simulink model "dyn_model"  (R2016b)
settings: Solver=VariableStepAuto  StartTime=0.0  StopTime=20  RelTol=1e-3
undefined symbols (not defined in the file or in its folder): D1, Delta
libraries: powerlib x29
settings Model: SimulationMode=accelerator  Creator=tinrabuzin  LastModifiedBy=tinrabuzin
settings SolverCC: ZeroCrossAlgorithm=Adaptive
settings DebuggingCC: UnconnectedInputMsg=none  UnconnectedOutputMsg=none  UnconnectedLineMsg=none

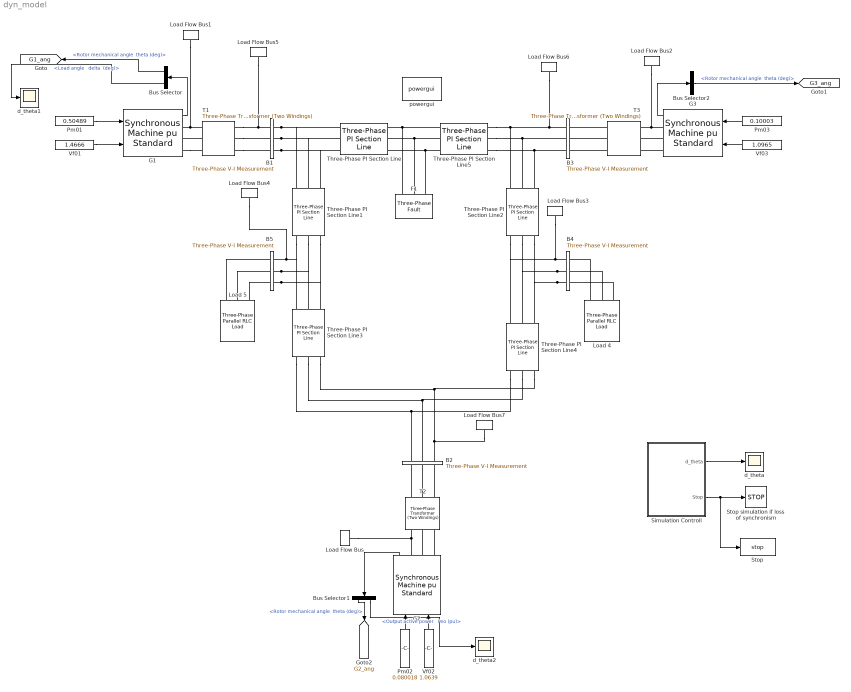
== system dyn_model ==
  B1 : powerlib/Measurements/Three-Phase V-I Measurement  VoltageMeasurement=phase-to-ground  SetLabelV=on  LabelV=Vabc_B1  Vpu=off  VpuLL=off  CurrentMeasurement=yes  SetLabelI=on  LabelI=Iabc_B1  Ipu=off  Pbase=100e6  Vbase=500e3  OutputType=Complex  PhasorSimulation=on  PSBequivalent=0
  B2 : powerlib/Measurements/Three-Phase V-I Measurement  VoltageMeasurement=phase-to-ground  SetLabelV=on  LabelV=Vabc_B2  Vpu=off  VpuLL=off  CurrentMeasurement=yes  SetLabelI=on  LabelI=Iabc_B2  Ipu=off  Pbase=100e6  Vbase=500e3  OutputType=Complex  PhasorSimulation=on  PSBequivalent=0
  B3 : powerlib/Measurements/Three-Phase V-I Measurement  VoltageMeasurement=phase-to-ground  SetLabelV=on  LabelV=Vabc_B3  Vpu=off  VpuLL=off  CurrentMeasurement=yes  SetLabelI=on  LabelI=Iabc_B3  Ipu=off  Pbase=100e6  Vbase=500e3  OutputType=Complex  PhasorSimulation=on  PSBequivalent=0
  B4 : powerlib/Measurements/Three-Phase V-I Measurement  VoltageMeasurement=phase-to-ground  SetLabelV=on  LabelV=Vabc_B4  Vpu=off  VpuLL=off  CurrentMeasurement=yes  SetLabelI=on  LabelI=Iabc_B4  Ipu=off  Pbase=100e6  Vbase=500e3  OutputType=Complex  PhasorSimulation=on  PSBequivalent=0
  B5 : powerlib/Measurements/Three-Phase V-I Measurement  VoltageMeasurement=phase-to-ground  SetLabelV=on  LabelV=Vabc_B5  Vpu=off  VpuLL=off  CurrentMeasurement=yes  SetLabelI=on  LabelI=Iabc_B5  Ipu=off  Pbase=100e6  Vbase=500e3  OutputType=Complex  PhasorSimulation=on  PSBequivalent=0
  Bus Selector : BusSelector  OutputSignals="Mechanical.Rotor mechanical angle  theta (deg),Load angle   delta  (deg)"
  Bus Selector1 : BusSelector  OutputSignals="Mechanical.Rotor mechanical angle  theta (deg),Output active power   Peo (pu)"
  Bus Selector2 : BusSelector  OutputSignals="Mechanical.Rotor mechanical angle  theta (deg)"
  F1 : powerlib/Elements/Three-Phase Fault  InitialStates=0  FaultA=on  FaultB=on  FaultC=on  GroundFault=on  SwitchTimes=[1 4.5005]  External=off  SwitchStatus=NaN  FaultResistance=0.0001  GroundResistance=0.0001  SnubberResistance=1e6  SnubberCapacitance=inf  Measurements=None
  G1 : powerlib/Machines/Synchronous Machine pu Standard  PresetModel=No  MechanicalLoad=Mechanical power Pm  ShowDetailedParameters=on  RotorType=Round  Units=per unit standard parameters  MeasurementBus=off  NominalParameters="[200E6  24000   50 ]"  Reactances1=[1.8 .3 .25 1.7 .55 .25 .2]  Reactances2=[ 1.305, 0.296, 0.252, 0.474, 0.243, 0.18 ]  dAxisTimeConstants=Open-circuit  qAxisTimeConstants=Open-circuit  TimeConstants1=[]  TimeConstants2=[8 .03 .4 .05]  TimeConstants3=[]  TimeConstants4=[]  TimeConstants5=[ 1.01, 0.053, 0.1 ]  TimeConstants6=[]  TimeConstants7=[]  TimeConstants8=[]  StatorResistance=0.0025  Mechanical=[ 6.5 0 2]  PolePairs=4  InitialConditions=[0 -53.1702 0.511213 0.511213 0.511213 -9.47522 -129.475 110.525 1.46662]  SetSaturation=off  Saturation=[0.6404,0.7127,0.8441,0.9214,0.9956,1.082,1.19,1.316,1.457;0.7,0.7698,0.8872,0.9466,0.9969,1.046,1.1,1.151,1.201]  LoadFlowParameters=[2 700000000 0 0 0]  TsPowergui=0  TsBlock=-1  IterativeModel=Trapezoidal non iterative  IterativeDiscreteModel=Trapezoidal non iterative  BusType=swing  Pref=700000000  Qref=0  Qmin=-Inf  Qmax=Inf  PLF=0  QLF=0
      settings: AttributesFormatString=\n\n
  G2 : powerlib/Machines/Synchronous Machine pu Standard  PresetModel=No  MechanicalLoad=Mechanical power Pm  ShowDetailedParameters=on  RotorType=Round  Units=per unit standard parameters  MeasurementBus=off  NominalParameters="[200E6  24000   50 ]"  Reactances1=[1.8 .3 .25 1.7 .55 .25 .2]  Reactances2=[ 1.305, 0.296, 0.252, 0.474, 0.243, 0.18 ]  dAxisTimeConstants=Open-circuit  qAxisTimeConstants=Open-circuit  TimeConstants1=[]  TimeConstants2=[8 .03 .4 .05]  TimeConstants3=[]  TimeConstants4=[]  TimeConstants5=[ 1.01, 0.053, 0.1 ]  TimeConstants6=[]  TimeConstants7=[]  TimeConstants8=[]  StatorResistance=0.0025  Mechanical=[ 6.5 0 2]  PolePairs=4  InitialConditions=[0 -91.9476 0.0854428 0.0854428 0.0854428 -29.8718 -149.872 90.1282 1.06392]  SetSaturation=off  Saturation=[0.6404,0.7127,0.8441,0.9214,0.9956,1.082,1.19,1.316,1.457;0.7,0.7698,0.8872,0.9466,0.9969,1.046,1.1,1.151,1.201]  LoadFlowParameters=[1 700000000 0 0 0]  TsPowergui=0  TsBlock=-1  IterativeModel=Trapezoidal non iterative  IterativeDiscreteModel=Trapezoidal non iterative  BusType=PQ  Pref=16000000  Qref=6000000  Qmin=-Inf  Qmax=Inf  PLF=0  QLF=0
      settings: AttributesFormatString=\n\n
  G3 : powerlib/Machines/Synchronous Machine pu Standard  PresetModel=No  MechanicalLoad=Mechanical power Pm  ShowDetailedParameters=on  RotorType=Round  Units=per unit standard parameters  MeasurementBus=off  NominalParameters="[200E6  24000   50 ]"  Reactances1=[1.8 .3 .25 1.7 .55 .25 .2]  Reactances2=[ 1.305, 0.296, 0.252, 0.474, 0.243, 0.18 ]  dAxisTimeConstants=Open-circuit  qAxisTimeConstants=Open-circuit  TimeConstants1=[]  TimeConstants2=[8 .03 .4 .05]  TimeConstants3=[]  TimeConstants4=[]  TimeConstants5=[ 1.01, 0.053, 0.1 ]  TimeConstants6=[]  TimeConstants7=[]  TimeConstants8=[]  StatorResistance=0.0025  Mechanical=[ 6.5 0 2]  PolePairs=4  InitialConditions=[0 -87.5459 0.109755 0.109755 0.109755 -30.8484 -150.848 89.1516 1.09649]  SetSaturation=off  Saturation=[0.6404,0.7127,0.8441,0.9214,0.9956,1.082,1.19,1.316,1.457;0.7,0.7698,0.8872,0.9466,0.9969,1.046,1.1,1.151,1.201]  LoadFlowParameters=[1 700000000 0 0 0]  TsPowergui=0  TsBlock=-1  IterativeModel=Trapezoidal non iterative  IterativeDiscreteModel=Trapezoidal non iterative  BusType=PV  Pref=20e6  Qref=0  Qmin=-Inf  Qmax=Inf  PLF=0  QLF=0
      settings: AttributesFormatString=\n\n
  Load 4 : powerlib/Elements/Three-Phase Parallel RLC Load  LConnTagsString=A|B|C  Configuration=Y (grounded)  NominalVoltage=220e3  Vabc=[1e3 1e3 1e3]  Vabcp=[1e3 1e3 1e3]  NominalFrequency=50  UnbalancedPower=off  ActivePower=70e6  InductivePower=1e6  CapacitivePower=0  Pabc=[10e3 9e3 11e3]  QLabc=[100 90 110]  QCabc=[100 90 110]  Pabcp=[10e3 9e3 11e3]  QLabcp=[100 90 110]  QCabcp=[100 90 110]  Measurements=None  LoadType=constant Z
  Load 5 : powerlib/Elements/Three-Phase Parallel RLC Load  LConnTagsString=A|B|C  Configuration=Y (grounded)  NominalVoltage=220e3  Vabc=[1e3 1e3 1e3]  Vabcp=[1e3 1e3 1e3]  NominalFrequency=50  UnbalancedPower=off  ActivePower=70e6  InductivePower=7e6  CapacitivePower=0  Pabc=[10e3 9e3 11e3]  QLabc=[100 90 110]  QCabc=[100 90 110]  Pabcp=[10e3 9e3 11e3]  QLabcp=[100 90 110]  QCabcp=[100 90 110]  Measurements=None  LoadType=constant Z
  Load Flow Bus : powerlib/Measurements/Load Flow Bus  LConnTagsString=a  Phases=single  Connectors=on one side  ID=BUS_2  Vbase=24e3  Vref=1  Vangle=0  VLF=1  VLFb=1  VLFc=1  angleLF=-9.316  angleLFb=0  angleLFc=0
  Load Flow Bus1 : powerlib/Measurements/Load Flow Bus  LConnTagsString=a  Phases=single  Connectors=on one side  ID=BUS_1  Vbase=24e3  Vref=1  Vangle=0  VLF=1  VLFb=1  VLFc=1  angleLF=0  angleLFb=0  angleLFc=0
  Load Flow Bus2 : powerlib/Measurements/Load Flow Bus  LConnTagsString=a  Phases=single  Connectors=on one side  ID=BUS_3  Vbase=24e3  Vref=1  Vangle=0  VLF=1  VLFb=1  VLFc=1  angleLF=-6.509  angleLFb=0  angleLFc=0
  Load Flow Bus3 : powerlib/Measurements/Load Flow Bus  LConnTagsString=a  Phases=single  Connectors=on one side  ID=BUS_4  Vbase=220e3  Vref=1  Vangle=0  VLF=0.9899  VLFb=1  VLFc=1  angleLF=16.45  angleLFb=0  angleLFc=0
  Load Flow Bus4 : powerlib/Measurements/Load Flow Bus  LConnTagsString=a  Phases=single  Connectors=on one side  ID=BUS_5  Vbase=220e3  Vref=1  Vangle=0  VLF=0.9784  VLFb=1  VLFc=1  angleLF=19.48  angleLFb=0  angleLFc=0
  Load Flow Bus5 : powerlib/Measurements/Load Flow Bus  LConnTagsString=a  Phases=single  Connectors=on one side  ID=BUS_11  Vbase=220e3  Vref=1  Vangle=0  VLF=0.9931  VLFb=1  VLFc=1  angleLF=27.1  angleLFb=0  angleLFc=0
  Load Flow Bus6 : powerlib/Measurements/Load Flow Bus  LConnTagsString=a  Phases=single  Connectors=on one side  ID=BUS_33  Vbase=220e3  Vref=1  Vangle=0  VLF=0.9957  VLFb=1  VLFc=1  angleLF=22.93  angleLFb=0  angleLFc=0
  Load Flow Bus7 : powerlib/Measurements/Load Flow Bus  LConnTagsString=a  Phases=single  Connectors=on one side  ID=BUS_22  Vbase=220e3  Vref=1  Vangle=0  VLF=0.9972  VLFb=1  VLFc=1  angleLF=20.24  angleLFb=0  angleLFc=0
  Pm01 : Constant  Value=0.50489
  Pm02 : Constant  Value=0.080018
  Pm03 : Constant  Value=0.10003
  Simulation Controll : Subsystem
  Stop : ToWorkspace  VariableName=stop  SaveFormat=Timeseries  SampleTime=-1
  Stop simulation if loss of synchronism : Stop
  T1 : powerlib/Elements/Three-Phase Transformer (Two Windings)  Winding1Connection=Delta (D1)  Winding2Connection=Yg  CoreType=Three single-phase transformers  SetSaturation=off  Hysteresis=off  DataFile='hysteresis'  SetInitialFlux=off  Measurements=None  UNITS=pu  NominalPower="[ 200e6   50 ]"  Winding1="[ 24e3  0   0]"  Winding2="[ 220e3  0   0.1]"  Rm=500  Lm=500  L0=0.5  Saturation="[ 0,0  ;  0.005,1.2  ;  1.0,1.4 ]"  InitialFluxes=[ 0.8 , -0.8 , 0.7 ]  MoreParameters=off  BreakLoop=off  DataType=off  TransfoNumber=0
  T2 : powerlib/Elements/Three-Phase Transformer (Two Windings)  Winding1Connection=Delta (D1)  Winding2Connection=Yg  CoreType=Three single-phase transformers  SetSaturation=off  Hysteresis=off  DataFile='hysteresis'  SetInitialFlux=off  Measurements=None  UNITS=pu  NominalPower="[ 200e6   50 ]"  Winding1="[ 24e3  0  0  ]"  Winding2="[ 220e3  0   0.1]"  Rm=500  Lm=500  L0=0.5  Saturation="[ 0,0  ;  0.005,1.2  ;  1.0,1.4 ]"  InitialFluxes=[ 0.8 , -0.8 , 0.7 ]  MoreParameters=off  BreakLoop=off  DataType=off  TransfoNumber=0
  T3 : powerlib/Elements/Three-Phase Transformer (Two Windings)  Winding1Connection=Delta (D1)  Winding2Connection=Yg  CoreType=Three single-phase transformers  SetSaturation=off  Hysteresis=off  DataFile='hysteresis'  SetInitialFlux=off  Measurements=None  UNITS=pu  NominalPower="[ 200e6   50 ]"  Winding1="[ 24e3 0   0  ]"  Winding2="[ 220e3  0   0.1 ]"  Rm=500  Lm=500  L0=0.5  Saturation="[ 0,0  ;  0.005,1.2  ;  1.0,1.4 ]"  InitialFluxes=[ 0.8 , -0.8 , 0.7 ]  MoreParameters=off  BreakLoop=off  DataType=off  TransfoNumber=0
  Three-Phase PI Section Line : powerlib/Elements/Three-Phase PI Section Line  LConnTagsString=a|b|c  RConnTagsString=A|B|C  Frequency=50  Resistances=[0 0]  Inductances="[48.4  4.1264e-1] / (2*pi*50)"  Capacitances=[12.74e-9 7.751e-9]  Length=1
  Three-Phase PI Section Line1 : powerlib/Elements/Three-Phase PI Section Line  LConnTagsString=a|b|c  RConnTagsString=A|B|C  Frequency=50  Resistances=[0 0]  Inductances="[96.8  4.1264e-1] / (2*pi*50)"  Capacitances=[12.74e-9 7.751e-9]  Length=1
  Three-Phase PI Section Line2 : powerlib/Elements/Three-Phase PI Section Line  LConnTagsString=a|b|c  RConnTagsString=A|B|C  Frequency=50  Resistances=[0 0]  Inductances="[96.8  4.1264e-1] / (2*pi*50)"  Capacitances=[12.74e-9 7.751e-9]  Length=1
  Three-Phase PI Section Line3 : powerlib/Elements/Three-Phase PI Section Line  LConnTagsString=a|b|c  RConnTagsString=A|B|C  Frequency=50  Resistances=[0 0]  Inductances=[242 4.1264e-1] / (2*pi*50)  Capacitances=[12.74e-9 7.751e-9]  Length=1
  Three-Phase PI Section Line4 : powerlib/Elements/Three-Phase PI Section Line  LConnTagsString=a|b|c  RConnTagsString=A|B|C  Frequency=50  Resistances=[0 0]  Inductances="[242  4.1264e-1] / (2*pi*50)"  Capacitances=[12.74e-9 7.751e-9]  Length=1
  Three-Phase PI Section Line5 : powerlib/Elements/Three-Phase PI Section Line  LConnTagsString=a|b|c  RConnTagsString=A|B|C  Frequency=50  Resistances=[0 0]  Inductances="[48.4  4.1264e-1] / (2*pi*50)"  Capacitances=[12.74e-9 7.751e-9]  Length=1
  Vf01 : Constant  Value=1.4666
  Vf02 : Constant  Value=1.0639
  Vf03 : Constant  Value=1.0965
  d_theta : Scope
  d_theta1 : Scope
  d_theta2 : Scope
  powergui : powerlib/powergui  Priority=1  SimulationMode=Phasor  SolverType=Tustin/Backward Euler (TBE)  SampleTime=50e-6  frequency=50  SPID=off  DisableSnubberDevices=off  DisableRonSwitches=off  DisableVfSwitches=off  SwTol=0  DisplayEquations=off  Interpol=off  ExternalGateDelay=off  methode=off  Ts=10  FunctionMessages=off  echomessages=off  HookPort=off  EnableUseOfTLC=off  x0status=blocks  frequencyindice=50  Pbase=100e6  ErrMax=0.0001  Iterations=300  UnitsV=kV  UnitsW=MW  buscounter=0  RestoreLinks=warning  ResistiveCurrentMeasurement=off  Frange=[0:2:500]  Ylog=off  Xlog=on  ShowGrid=off  save=off  variable=ZData  structure=0  ZoomFFT=off  StartTime=0.0  cycles=1  DisplayStyle=1  fundamental=60  FreqAxis=off  MaxFrequency=1000  frequencyindicesteady=1  RmsSteady=1  display=off
  tag scope: G1_ang=global, G2_ang=global, G3_ang=global
  wires:
  Pm01/1 -> G1/1
  Vf01/1 -> G1/2
  Vf03/1 -> G3/2
  Pm03/1 -> G3/1
  Vf02/1 -> G2/2
  Pm02/1 -> G2/1
  G1/1 -> Bus Selector/1
  Bus Selector/1 -> [G1_ang]  "<Rotor mechanical angle  theta (deg)>"
  G3/1 -> Bus Selector2/1
  Bus Selector2/1 -> [G3_ang]  "<Rotor mechanical angle  theta (deg)>"
  G2/1 -> Bus Selector1/1
  Bus Selector1/1 -> [G2_ang]  "<Rotor mechanical angle  theta (deg)>"
  Simulation Controll/1(d_theta) -> d_theta/1
  Simulation Controll/2(Stop) -> Stop simulation if loss of synchronism/1, Stop/1
  Bus Selector/2 -> d_theta1/1  "<Load angle   delta  (deg)>"
  Bus Selector1/2 -> d_theta2/1  "<Output active power   Peo (pu)>"
  connections:
  B1/RConn1 -- Three-Phase PI Section Line1/LConn1 -- Three-Phase PI Section Line/LConn1
  B1/RConn2 -- Three-Phase PI Section Line1/LConn2 -- Three-Phase PI Section Line/LConn2
  B1/RConn3 -- Three-Phase PI Section Line1/LConn3 -- Three-Phase PI Section Line/LConn3
  Three-Phase PI Section Line2/LConn1 -- Three-Phase PI Section Line5/RConn1 -- B3/RConn3 -- Load Flow Bus6/LConn1
  Three-Phase PI Section Line2/LConn2 -- B3/RConn2 -- Three-Phase PI Section Line5/RConn2
  Three-Phase PI Section Line2/LConn3 -- B3/RConn1 -- Three-Phase PI Section Line5/RConn3
  Three-Phase PI Section Line3/LConn1 -- Three-Phase PI Section Line1/RConn1 -- Load Flow Bus4/LConn1 -- B5/LConn3
  B5/LConn2 -- Three-Phase PI Section Line3/LConn2 -- Three-Phase PI Section Line1/RConn2
  B5/LConn1 -- Three-Phase PI Section Line3/LConn3 -- Three-Phase PI Section Line1/RConn3
  Three-Phase PI Section Line4/LConn1 -- Three-Phase PI Section Line2/RConn1 -- Load Flow Bus3/LConn1 -- B4/RConn3
  B4/RConn2 -- Three-Phase PI Section Line4/LConn2 -- Three-Phase PI Section Line2/RConn2
  B4/RConn1 -- Three-Phase PI Section Line4/LConn3 -- Three-Phase PI Section Line2/RConn3
  Three-Phase PI Section Line4/RConn1 -- B2/LConn3 -- Three-Phase PI Section Line3/RConn1
  Three-Phase PI Section Line4/RConn2 -- Three-Phase PI Section Line3/RConn2 -- B2/LConn2
  Three-Phase PI Section Line4/RConn3 -- Three-Phase PI Section Line3/RConn3 -- Load Flow Bus7/LConn1 -- B2/LConn1
  Load 5/LConn1 -- B5/RConn3
  Load 5/LConn2 -- B5/RConn2
  Load 5/LConn3 -- B5/RConn1
  Load 4/LConn1 -- B4/LConn3
  Load 4/LConn2 -- B4/LConn2
  Load 4/LConn3 -- B4/LConn1
  T1/RConn1 -- Load Flow Bus5/LConn1 -- B1/LConn1
  T1/RConn2 -- B1/LConn2
  T1/RConn3 -- B1/LConn3
  T3/RConn1 -- B3/LConn3
  T3/RConn2 -- B3/LConn2
  T3/RConn3 -- B3/LConn1
  T2/RConn1 -- B2/RConn3
  T2/RConn2 -- B2/RConn2
  T2/RConn3 -- B2/RConn1
  G1/RConn1 -- T1/LConn1 -- Load Flow Bus1/LConn1
  T1/LConn2 -- G1/RConn2
  G1/RConn3 -- T1/LConn3
  G2/RConn1 -- Load Flow Bus/LConn1 -- T2/LConn1
  G2/RConn2 -- T2/LConn2
  G2/RConn3 -- T2/LConn3
  G3/RConn1 -- Load Flow Bus2/LConn1 -- T3/LConn1
  G3/RConn2 -- T3/LConn2
  G3/RConn3 -- T3/LConn3
  Three-Phase PI Section Line5/LConn1 -- F1/LConn1 -- Three-Phase PI Section Line/RConn1
  Three-Phase PI Section Line5/LConn2 -- F1/LConn2 -- Three-Phase PI Section Line/RConn2
  Three-Phase PI Section Line5/LConn3 -- F1/LConn3 -- Three-Phase PI Section Line/RConn3

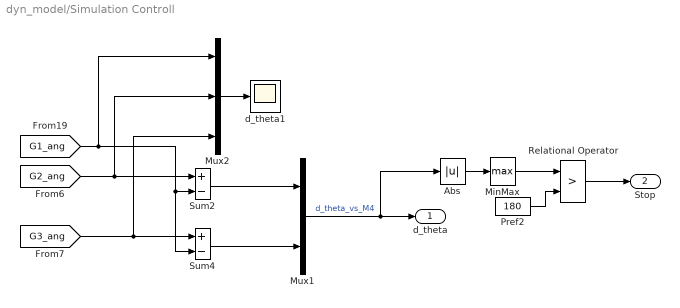
== system dyn_model/Simulation Controll ==
  Abs : Abs  SaturateOnIntegerOverflow=on
  MinMax : MinMax  Function=max  SaturateOnIntegerOverflow=on  InputSameDT=on
  Mux1 : Mux  Inputs=2
  Mux2 : Mux  Inputs=3
  Pref2 : Constant  Value=180
  Relational Operator : RelationalOperator  Operator=>  RndMeth=Nearest  InputSameDT=on
  Sum2 : Sum  Inputs=+-  SaturateOnIntegerOverflow=on  InputSameDT=on  OutDataTypeStr=Inherit: Same as first input
  Sum4 : Sum  Inputs=+-  SaturateOnIntegerOverflow=on  InputSameDT=on  OutDataTypeStr=Inherit: Same as first input
  d_theta1 : Scope
  d_theta : Outport
  Stop : Outport  Port=2
  wires:
  Mux1/1 -> d_theta/1, Abs/1  "d_theta_vs_M4"
  Abs/1 -> MinMax/1
  Pref2/1 -> Relational Operator/2
  MinMax/1 -> Relational Operator/1
  Relational Operator/1 -> Stop/1
  Sum2/1 -> Mux1/1
  Sum4/1 -> Mux1/2
  [G2_ang] -> Mux2/2, Sum2/1
  [G3_ang] -> Mux2/3, Sum4/1
  [G1_ang] -> Mux2/1, Sum4/2, Sum2/2
  Mux2/1 -> d_theta1/1
